simulink model "Model"  (R2019a)
settings: Solver=VariableStepAuto  StartTime=0.0  StopTime=10.0  RelTol=1e-3
model workspace (MAT data in the model file):
  Var = 0
values from neighbouring files (symbols this model uses):
  K = zeros(3,2)    [Task4.m]
settings Model: OrderedModelArguments=off  Creator=ted03  LastModifiedBy=ted03

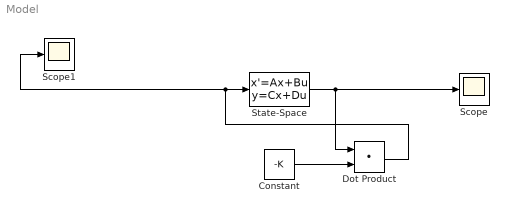
== system Model ==
  Constant : Constant  Value=-K
  Dot Product : DotProduct  InputSameDT=on  OutDataTypeStr=Inherit: Inherit via internal rule
  Scope : Scope
  Scope1 : Scope
  State-Space : StateSpace  A=[0,1;0,0]  B=[0;1]  C=[1,0;0,1]  D=[0;0]  InitialCondition=[-10;-10]
  wires:
  State-Space/1 -> Dot Product/1, Scope/1
  Constant/1 -> Dot Product/2
  Dot Product/1 -> Scope1/1, State-Space/1
